simulink model "spring"  (R2020b)
settings: Solver=VariableStepAuto  StartTime=0.0  StopTime=10.0  RelTol=1e-3
undefined symbols (not defined in the file): b, k1, k2, m1, m2
settings Model: Creator=Manasi  LastModifiedBy=Manasi

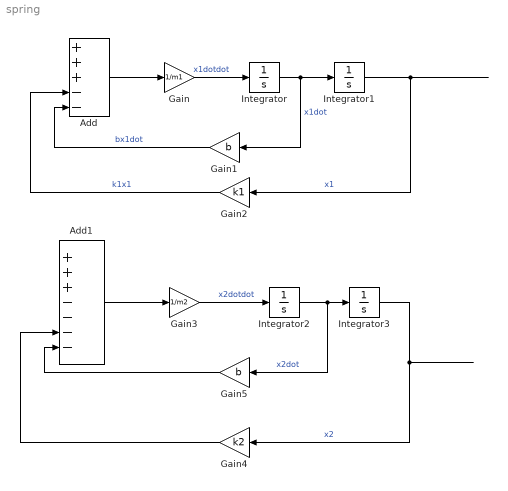
== system spring ==
  Add : Sum  Inputs=+++--
  Add1 : Sum  Inputs=+++----
  Gain : Gain  Gain=1/m1
  Gain1 : Gain  Gain=b
  Gain2 : Gain  Gain=k1
  Gain3 : Gain  Gain=1/m2
  Gain4 : Gain  Gain=k2
  Gain5 : Gain  Gain=b
  Integrator{,1..3} (4 alike) : Integrator
  wires:
  Add/1 -> Gain/1
  Gain/1 -> Integrator/1  "x1dotdot"
  Integrator/1 -> Gain1/1, Integrator1/1  "x1dot"
  Integrator1/1 -> Gain2/1  "x1"
  Gain1/1 -> Add/5  "bx1dot"
  Gain2/1 -> Add/4  "k1x1"
  Add1/1 -> Gain3/1
  Gain3/1 -> Integrator2/1  "x2dotdot"
  Integrator2/1 -> Gain5/1, Integrator3/1  "x2dot"
  Integrator3/1 -> Gain4/1  "x2"
  Gain5/1 -> Add1/7
  Gain4/1 -> Add1/6
